simulink model "virtual_world"  (R2020b)
settings: Solver=FixedStepAuto  StartTime=0.0  StopTime=60  FixedStep=0.05  RelTol=1e-3
model workspace (MAT data in the model file):
  Delay = 4
undefined symbols (not defined in the file): serial
libraries: instrumentlib x6, simulink x3
settings Model: SimulationMode=external  Creator=Mostafa  LastModifiedBy=Mostafa
settings SFSimCC: SimTargetLang=C++
settings RTWCC: Description=Simulink Desktop Real-Time  SystemTargetFile=sldrt.tlc  TemplateMakefile=sldrt.tmf  TargetLang=C++  RTWCompilerOptimization=on
settings CodeAppCC: MaxIdLength=95
settings SimulinkDesktopRealTimeCC: TargetPreCompLibLocation=C:\Program Files\Polyspace\R2020b\toolbox\sldrt\lib\win64  TargetLangStandard=C++03 (ISO)

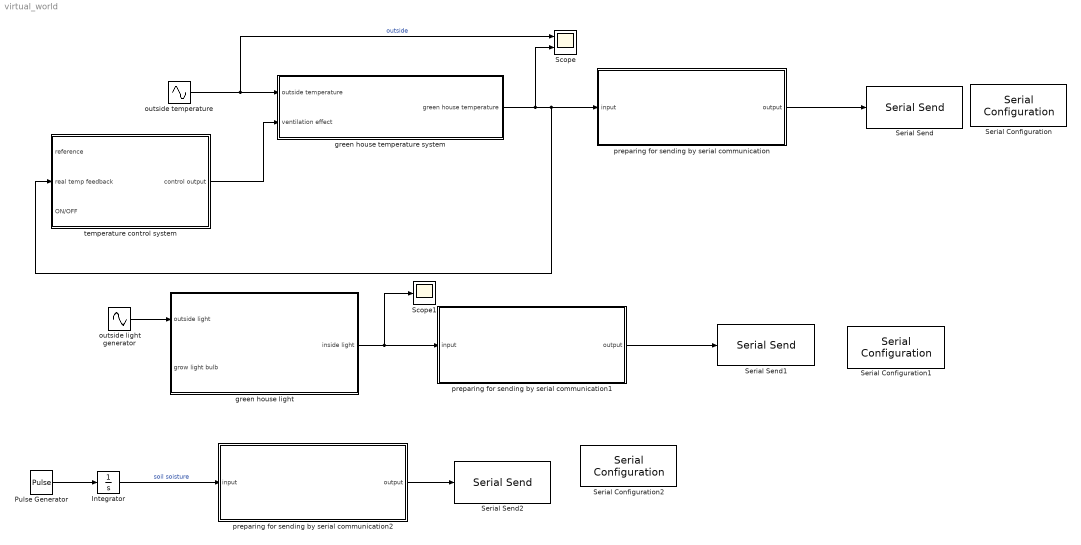
== system virtual_world ==
  Integrator : Integrator
  Pulse Generator : DiscretePulseGenerator  PulseType=Time based  Period=10  PulseWidth=50
  Scope : Scope  NumInputPorts=2
  Scope1 : Scope
  Serial Configuration : instrumentlib/Serial Configuration  Priority=-200000  ComPortMenu=COM20  ComPort=COM20  ObjConstructor=serial('COM20');  BaudRate=9600  DataBits=8  Parity=none  StopBits=1  FlowControl=none  Timeout=10  ByteOrder=LittleEndian
  Serial Configuration1 : instrumentlib/Serial Configuration  Priority=-200000  ComPortMenu=COM30  ComPort=COM30  ObjConstructor=serial('COM30');  BaudRate=9600  DataBits=8  Parity=none  StopBits=1  FlowControl=none  Timeout=10  ByteOrder=LittleEndian
  Serial Configuration2 : instrumentlib/Serial Configuration  Priority=-200000  ComPortMenu=COM40  ComPort=COM40  ObjConstructor=serial('COM40');  BaudRate=9600  DataBits=8  Parity=none  StopBits=1  FlowControl=none  Timeout=10  ByteOrder=LittleEndian
  Serial Send : instrumentlib/Serial Send  ComPortMenu=COM20  ComPort=COM20  ObjConstructor=serial('COM20');  Terminator=<none>  EnableBlockingMode=on
  Serial Send1 : instrumentlib/Serial Send  ComPortMenu=COM30  ComPort=COM30  ObjConstructor=serial('COM30');  Terminator=<none>  EnableBlockingMode=on
  Serial Send2 : instrumentlib/Serial Send  ComPortMenu=COM40  ComPort=COM40  ObjConstructor=serial('COM40');  Terminator=<none>  EnableBlockingMode=on
  green house light : Subsystem
  green house temperature system : Subsystem
  outside light generator : Sin  Amplitude=50  Bias=50  Frequency=2*pi/40  SampleTime=0
  outside temperature : Sin  Amplitude=5  Bias=25  Frequency=2*pi/40  SampleTime=0
  preparing for sending by serial communication : Subsystem
  preparing for sending by serial communication1 : Subsystem
  preparing for sending by serial communication2 : Subsystem
  temperature control system : Subsystem
  wires:
  outside temperature/1 -> Scope/1, green house temperature system/1(outside temperature)  "outside"
  temperature control system/1(control output) -> green house temperature system/2(ventilation effect)
  outside light generator/1 -> green house light/1(outside light)
  preparing for sending by serial communication/1(output) -> Serial Send/1
  preparing for sending by serial communication1/1(output) -> Serial Send1/1
  green house light/1(inside light) -> Scope1/1, preparing for sending by serial communication1/1(input)
  green house temperature system/1(green house temperature) -> preparing for sending by serial communication/1(input), temperature control system/2(real temp feedback), Scope/2
  preparing for sending by serial communication2/1(output) -> Serial Send2/1
  Integrator/1 -> preparing for sending by serial communication2/1(input)  "soil soisture"
  Pulse Generator/1 -> Integrator/1

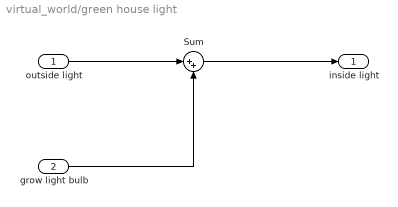
== system virtual_world/green house light ==
  outside light : Inport
  grow light bulb : Inport  Port=2
  Sum : Sum  Inputs=|++
  inside light : Outport
  wires:
  grow light bulb/1 -> Sum/2
  outside light/1 -> Sum/1
  Sum/1 -> inside light/1

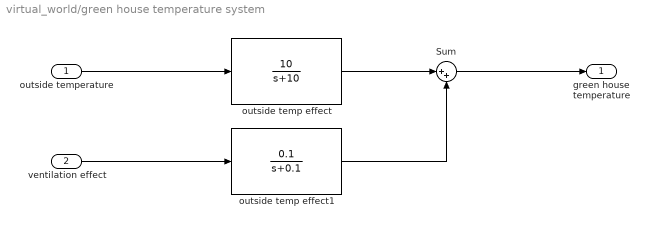
== system virtual_world/green house temperature system ==
  outside temperature : Inport
  ventilation effect : Inport  Port=2
  Sum : Sum  Inputs=|++
  outside temp effect : TransferFcn  Numerator=[10]  Denominator=[1 10]
  outside temp effect1 : TransferFcn  Numerator=[0.1]  Denominator=[1 0.1]
  green house temperature : Outport
  wires:
  outside temperature/1 -> outside temp effect/1
  outside temp effect/1 -> Sum/1
  Sum/1 -> green house temperature/1
  outside temp effect1/1 -> Sum/2
  ventilation effect/1 -> outside temp effect1/1

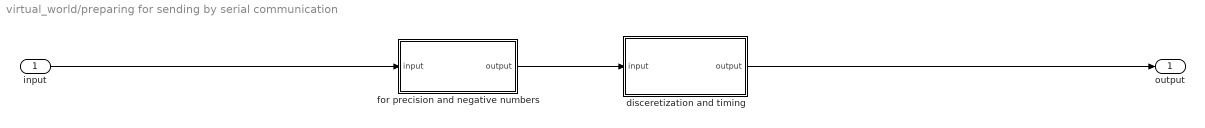
== system virtual_world/preparing for sending by serial communication ==
  input : Inport
  disceretization and timing : Subsystem
  for precision and negative numbers : Subsystem
  output : Outport
  wires:
  for precision and negative numbers/1(output) -> disceretization and timing/1(input)
  input/1 -> for precision and negative numbers/1(input)
  disceretization and timing/1(output) -> output/1

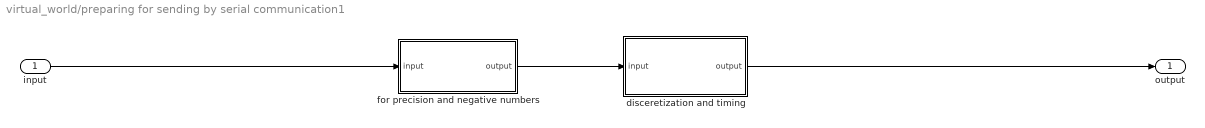
== system virtual_world/preparing for sending by serial communication1 ==
  input : Inport
  disceretization and timing : Subsystem
  for precision and negative numbers : Subsystem
  output : Outport
  wires:
  disceretization and timing/1(output) -> output/1
  input/1 -> for precision and negative numbers/1(input)
  for precision and negative numbers/1(output) -> disceretization and timing/1(input)

== system virtual_world/preparing for sending by serial communication2 ==
  input : Inport
  disceretization and timing : Subsystem
  for precision and negative numbers : Subsystem
  output : Outport
  wires:
  for precision and negative numbers/1(output) -> disceretization and timing/1(input)
  input/1 -> for precision and negative numbers/1(input)
  disceretization and timing/1(output) -> output/1

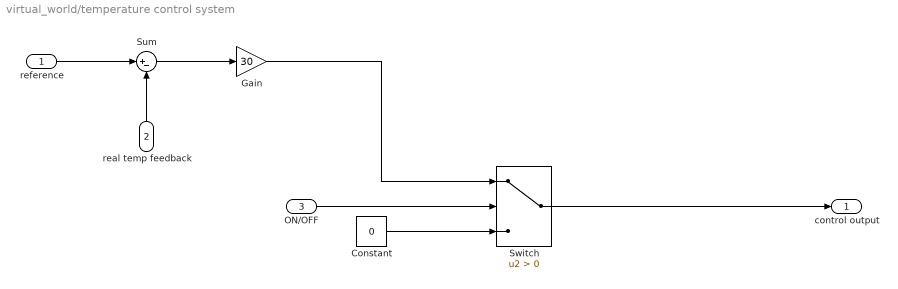
== system virtual_world/temperature control system ==
  reference : Inport
  real temp feedback : Inport  Port=2
  ON/OFF : Inport  Port=3
  Constant : Constant  Value=0
  Gain : Gain  Gain=30
  Sum : Sum  Inputs=|+-
  Switch : Switch  Criteria=u2 > Threshold
  control output : Outport
  wires:
  ON/OFF/1 -> Switch/2
  Switch/1 -> control output/1
  Constant/1 -> Switch/3
  Sum/1 -> Gain/1
  reference/1 -> Sum/1
  real temp feedback/1 -> Sum/2
  Gain/1 -> Switch/1

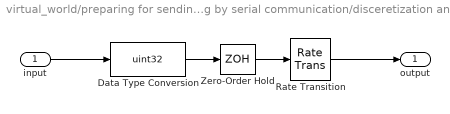
== system virtual_world/preparing for sending by serial communication/disceretization and timing ==
  input : Inport
  Data Type Conversion : DataTypeConversion  OutDataTypeStr=uint32
  Rate Transition : RateTransition  OutPortSampleTime=Delay
  Zero-Order Hold : ZeroOrderHold  SampleTime=Delay
  output : Outport
  wires:
  Zero-Order Hold/1 -> Rate Transition/1
  input/1 -> Data Type Conversion/1
  Data Type Conversion/1 -> Zero-Order Hold/1
  Rate Transition/1 -> output/1

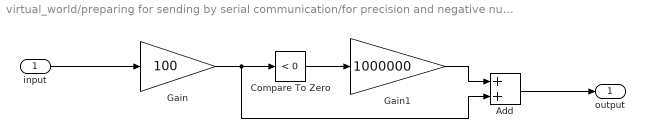
== system virtual_world/preparing for sending by serial communication/for precision and negative numbers ==
  input : Inport
  Add : Sum
  Compare To Zero : simulink/Logic and Bit Operations/Compare To Zero  relop=<  OutDataTypeStr=boolean
  Gain : Gain  Gain=100
  Gain1 : Gain  Gain=1000000  ParamDataTypeStr=double  OutDataTypeStr=double
  output : Outport
  wires:
  Compare To Zero/1 -> Gain1/1
  Add/1 -> output/1
  Gain1/1 -> Add/1
  Gain/1 -> Add/2, Compare To Zero/1
  input/1 -> Gain/1

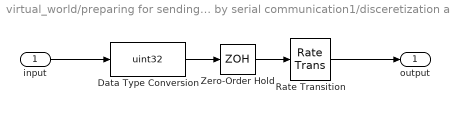
== system virtual_world/preparing for sending by serial communication1/disceretization and timing ==
  input : Inport
  Data Type Conversion : DataTypeConversion  OutDataTypeStr=uint32
  Rate Transition : RateTransition  OutPortSampleTime=Delay
  Zero-Order Hold : ZeroOrderHold  SampleTime=Delay
  output : Outport
  wires:
  Rate Transition/1 -> output/1
  Data Type Conversion/1 -> Zero-Order Hold/1
  input/1 -> Data Type Conversion/1
  Zero-Order Hold/1 -> Rate Transition/1

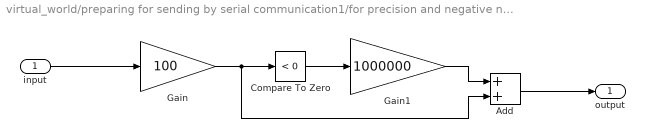
== system virtual_world/preparing for sending by serial communication1/for precision and negative numbers ==
  input : Inport
  Add : Sum
  Compare To Zero : simulink/Logic and Bit Operations/Compare To Zero  relop=<  OutDataTypeStr=boolean
  Gain : Gain  Gain=100
  Gain1 : Gain  Gain=1000000  ParamDataTypeStr=double  OutDataTypeStr=double
  output : Outport
  wires:
  input/1 -> Gain/1
  Gain/1 -> Compare To Zero/1, Add/2
  Gain1/1 -> Add/1
  Add/1 -> output/1
  Compare To Zero/1 -> Gain1/1

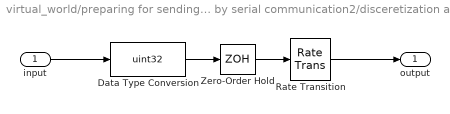
== system virtual_world/preparing for sending by serial communication2/disceretization and timing ==
  input : Inport
  Data Type Conversion : DataTypeConversion  OutDataTypeStr=uint32
  Rate Transition : RateTransition  OutPortSampleTime=Delay
  Zero-Order Hold : ZeroOrderHold  SampleTime=Delay
  output : Outport
  wires:
  Zero-Order Hold/1 -> Rate Transition/1
  input/1 -> Data Type Conversion/1
  Data Type Conversion/1 -> Zero-Order Hold/1
  Rate Transition/1 -> output/1

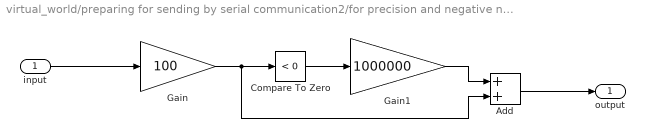
== system virtual_world/preparing for sending by serial communication2/for precision and negative numbers ==
  input : Inport
  Add : Sum
  Compare To Zero : simulink/Logic and Bit Operations/Compare To Zero  relop=<  OutDataTypeStr=boolean
  Gain : Gain  Gain=100
  Gain1 : Gain  Gain=1000000  ParamDataTypeStr=double  OutDataTypeStr=double
  output : Outport
  wires:
  Compare To Zero/1 -> Gain1/1
  Add/1 -> output/1
  Gain1/1 -> Add/1
  Gain/1 -> Add/2, Compare To Zero/1
  input/1 -> Gain/1
